simulink library "lib_FDM"  (R2019b)
settings: Solver=VariableStepAuto  StartTime=0.0  StopTime=10.0  RelTol=1e-3
values from neighbouring files (symbols this model uses):
  d = config.d_m    [computeTF.m]
undefined symbols (not defined in the file or in its folder): c_b_WGS, c_flat, c_grav, c_rot, c_rsma, Cd0, Cdcl, Cdcl2, Cl0, Cla, Cld, Cma, Cmd, Cmq, Cnb, Cnd, Cnr, Cra, Crd, Crp, Cy0, Cyb, Cyd, dmdt, Earth, HIL_Data, InitThrust, launchPos, me, mf, mp, Sref, tb, TF, theta0, WGS84
libraries: simulink_extras x14, $bdroot x7, simulink x5, lib_Fin_Deflections x3, aerolibasang x2, sharedtransform x1, aerolibtransform2 x1, aerolibbdyn x1, aerolibatmos2 x1, aerolibutil x1, aerolib6dof2 x1
(part 6 of 8)

== system lib_FDM/FDM/FDM_Sophisticated/environment/atmosphere_static_ISO_2533/tmp_and_pressure_ISO_2533/static_Temperature ==
  Tmp_ref : Inport
  h_geop : Inport  Port=2
  h_geop_ref : Inport  Port=3
  Add : Sum
  Product : Product
  Subtract : Sum  Inputs=+-
  Tmp_gradient_tropo : Constant  Value=HIL_Data.FDM.soph.bus2.c_be
  Tmp : Outport  VectorParamsAs1DForOutWhenUnconnected=off
  wires:
  h_geop_ref/1 -> Subtract/2
  h_geop/1 -> Subtract/1
  Tmp_ref/1 -> Add/1
  Add/1 -> Tmp/1  "Tmp"
  Product/1 -> Add/2
  Tmp_gradient_tropo/1 -> Product/1
  Subtract/1 -> Product/2

== system lib_FDM/FDM/FDM_Sophisticated/environment/atmosphere_static_ISO_2533/tmp_and_pressure_ISO_2533/static_pressure ==
  h_geop_ref : Inport
  h_geop : Inport  Port=2
  Tmp_ref : Inport  Port=3
  pa_ref : Inport  Port=4
  Add : Sum
  Constant1 : Constant
  Divide : Product  Inputs=*/*
  Math Function : Math  Operator=pow  SaturateOnIntegerOverflow=on
  Product : Product
  Subtract : Sum  Inputs=-+
  Tmp_gradient_tropo : Constant  Value=HIL_Data.FDM.soph.bus2.c_be
  pressure_exponent : Constant  Value=HIL_Data.FDM.soph.bus2.c_pe
  pa : Outport  VectorParamsAs1DForOutWhenUnconnected=off
  wires:
  Tmp_gradient_tropo/1 -> Divide/3
  Product/1 -> pa/1  "pa"
  Constant1/1 -> Add/1
  Subtract/1 -> Divide/1
  Math Function/1 -> Product/1
  pa_ref/1 -> Product/2
  Add/1 -> Math Function/1
  Tmp_ref/1 -> Divide/2
  h_geop_ref/1 -> Subtract/1
  Divide/1 -> Add/2
  h_geop/1 -> Subtract/2
  pressure_exponent/1 -> Math Function/2

== system lib_FDM/FDM/FDM_Sophisticated/gravity/launch_rail/initial_altitude/trafo_E_to_geodetic ==
  note: Inputs [size]:
      |
      | position_E [3]
  note: Outputs [size]:
      |
      | geodetic longitude [1]
      | geodetic latitude [1]
      | geodetic altitude [1]
  pBEE : Inport
  Geodetic_altitude : Subsystem
  Geodetic_latitude : Subsystem
  Selector1 : Selector  IndexMode=Zero-based  InputPortWidth=3  IndexOptions=Index vector (dialog)  Indices=1  OutputSizes=1
  Selector2 : Selector  IndexMode=Zero-based  InputPortWidth=3  IndexOptions=Index vector (dialog)  Indices=0  OutputSizes=1
  Trigonometric Function1 : Trigonometry  Operator=atan2
  c_flat : Constant  Value=c_flat
  c_rsma : Constant  Value=c_rsma
  lon : Outport  VectorParamsAs1DForOutWhenUnconnected=off
  lat : Outport  Port=2  VectorParamsAs1DForOutWhenUnconnected=off
  alt : Outport  Port=3  VectorParamsAs1DForOutWhenUnconnected=off
  wires:
  pBEE/1 -> Geodetic_altitude/1(pBEE), Geodetic_latitude/1(pBEE), Selector2/1, Selector1/1  "pBEE"
  Trigonometric Function1/1 -> lon/1  "lon"
  Geodetic_altitude/1(alt) -> alt/1
  Geodetic_latitude/1(lat) -> lat/1, Geodetic_altitude/4(lat)
  Selector2/1 -> Trigonometric Function1/2  "pBEE_x"
  Selector1/1 -> Trigonometric Function1/1  "pBEE_y"
  c_rsma/1 -> Geodetic_altitude/2(c_rsma), Geodetic_latitude/2(c_rsma)  "c_rsma"
  c_flat/1 -> Geodetic_latitude/3(c_flat), Geodetic_altitude/3(c_flat)  "c_flat"

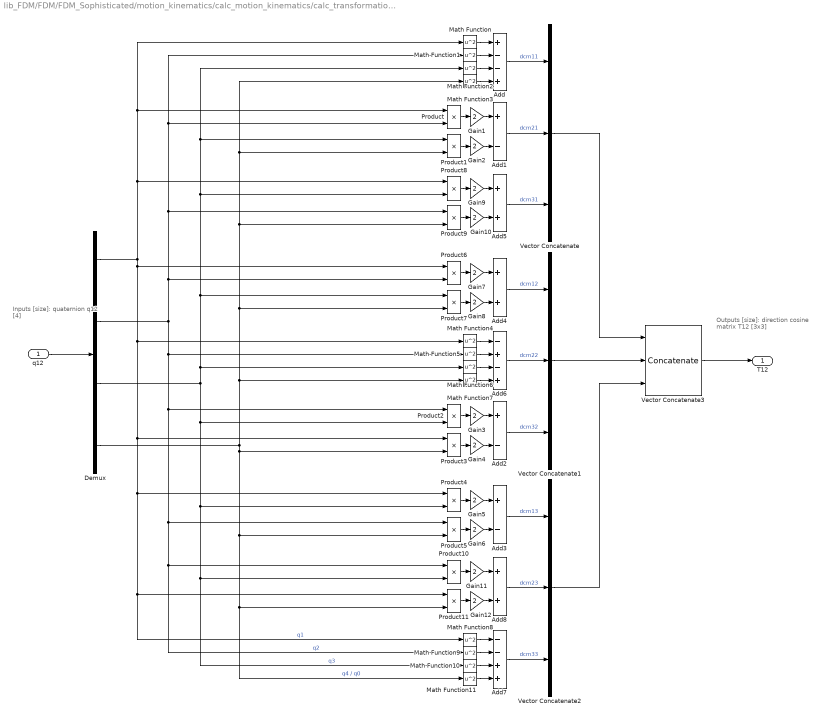
== system lib_FDM/FDM/FDM_Sophisticated/motion_kinematics/calc_motion_kinematics/calc_transformation_matrix/T12_from_q1 ==
  note: Outputs [size]:
      |
      | direction cosine matrix T12 [3x3]
  note: Inputs [size]:
      |
      | quaternion q12 [4]
  q12 : Inport  PortDimensions=4
  Add : Sum  Inputs=+--+
  Add1 : Sum  Inputs=+-
  Add2 : Sum  Inputs=+-
  Add3 : Sum  Inputs=+-
  Add4 : Sum
  Add5 : Sum
  Add6 : Sum  Inputs=-+-+
  Add7 : Sum  Inputs=--++
  Add8 : Sum
  Demux : Demux
  Gain{1..12} (12 alike) : Gain  Gain=2
  Math Function{,1..11} (12 alike) : Math  Operator=square  SaturateOnIntegerOverflow=on
  Product{,1..11} (12 alike) : Product
  Vector Concatenate : Concatenate  NumInputs=3
  Vector Concatenate1 : Concatenate  NumInputs=3
  Vector Concatenate2 : Concatenate  NumInputs=3
  Vector Concatenate3 : Concatenate  NumInputs=3  Mode=Multidimensional array  ConcatenateDimension=2
  T12 : Outport  PortDimensions=[3 3]  VectorParamsAs1DForOutWhenUnconnected=off
  wires:
  q12/1 -> Demux/1
  Demux/1 -> Product8/1, Product/1, Math Function/1, Product3/1, Product4/1, Product11/1, Math Function8/1, Math Function4/1, Product6/1  "q1"
  Demux/2 -> Product2/1, Product5/1, Product10/1, Math Function9/1, Math Function5/1, Product6/2, Product9/1, Product/2, Math Function1/1  "q2"
  Demux/3 -> Product2/2, Product4/2, Math Function10/1, Product10/2, Math Function6/1, Product7/1, Product8/2, Product1/1, Math Function2/1  "q3"
  Demux/4 -> Math Function7/1, Product7/2, Product9/2, Product1/2, Math Function3/1, Product5/2, Math Function11/1, Product11/2, Product3/2  "q4 / q0"
  Vector Concatenate3/1 -> T12/1
  Vector Concatenate/1 -> Vector Concatenate3/1
  Vector Concatenate2/1 -> Vector Concatenate3/3
  Vector Concatenate1/1 -> Vector Concatenate3/2
  Add/1 -> Vector Concatenate/1  "dcm11"
  Add1/1 -> Vector Concatenate/2  "dcm21"
  Add5/1 -> Vector Concatenate/3  "dcm31"
  Add4/1 -> Vector Concatenate1/1  "dcm12"
  Add6/1 -> Vector Concatenate1/2  "dcm22"
  Add2/1 -> Vector Concatenate1/3  "dcm32"
  Add3/1 -> Vector Concatenate2/1  "dcm13"
  Add8/1 -> Vector Concatenate2/2  "dcm23"
  Add7/1 -> Vector Concatenate2/3  "dcm33"
  Math Function/1 -> Add/1
  Math Function1/1 -> Add/2
  Math Function2/1 -> Add/3
  Math Function3/1 -> Add/4
  Product/1 -> Gain1/1
  Product1/1 -> Gain2/1
  Gain1/1 -> Add1/1
  Gain2/1 -> Add1/2
  Gain4/1 -> Add2/2
  Gain3/1 -> Add2/1
  Product3/1 -> Gain4/1
  Product2/1 -> Gain3/1
  Gain6/1 -> Add3/2
  Gain5/1 -> Add3/1
  Product5/1 -> Gain6/1
  Product4/1 -> Gain5/1
  Gain8/1 -> Add4/2
  Gain7/1 -> Add4/1
  Product7/1 -> Gain8/1
  Product6/1 -> Gain7/1
  Gain10/1 -> Add5/2
  Gain9/1 -> Add5/1
  Product9/1 -> Gain10/1
  Product8/1 -> Gain9/1
  Math Function6/1 -> Add6/3
  Math Function7/1 -> Add6/4
  Math Function5/1 -> Add6/2
  Math Function4/1 -> Add6/1
  Math Function10/1 -> Add7/3
  Math Function11/1 -> Add7/4
  Math Function9/1 -> Add7/2
  Math Function8/1 -> Add7/1
  Gain12/1 -> Add8/2
  Gain11/1 -> Add8/1
  Product11/1 -> Gain12/1
  Product10/1 -> Gain11/1

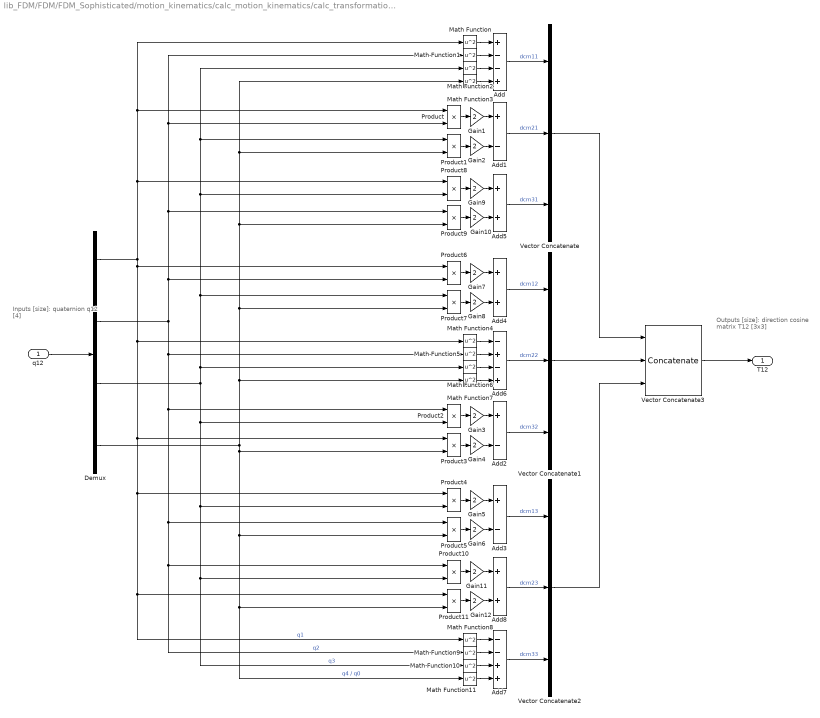
== system lib_FDM/FDM/FDM_Sophisticated/motion_kinematics/calc_motion_kinematics/calc_transformation_matrix/T12_from_q12 ==
  note: Outputs [size]:
      |
      | direction cosine matrix T12 [3x3]
  note: Inputs [size]:
      |
      | quaternion q12 [4]
  q12 : Inport  PortDimensions=4
  Add : Sum  Inputs=+--+
  Add1 : Sum  Inputs=+-
  Add2 : Sum  Inputs=+-
  Add3 : Sum  Inputs=+-
  Add4 : Sum
  Add5 : Sum
  Add6 : Sum  Inputs=-+-+
  Add7 : Sum  Inputs=--++
  Add8 : Sum
  Demux : Demux
  Gain{1..12} (12 alike) : Gain  Gain=2
  Math Function{,1..11} (12 alike) : Math  Operator=square  SaturateOnIntegerOverflow=on
  Product{,1..11} (12 alike) : Product
  Vector Concatenate : Concatenate  NumInputs=3
  Vector Concatenate1 : Concatenate  NumInputs=3
  Vector Concatenate2 : Concatenate  NumInputs=3
  Vector Concatenate3 : Concatenate  NumInputs=3  Mode=Multidimensional array  ConcatenateDimension=2
  T12 : Outport  PortDimensions=[3 3]  VectorParamsAs1DForOutWhenUnconnected=off
  wires:
  q12/1 -> Demux/1
  Demux/1 -> Product8/1, Product/1, Math Function/1, Product3/1, Product4/1, Product11/1, Math Function8/1, Math Function4/1, Product6/1  "q1"
  Demux/2 -> Product2/1, Product5/1, Product10/1, Math Function9/1, Math Function5/1, Product6/2, Product9/1, Product/2, Math Function1/1  "q2"
  Demux/3 -> Product2/2, Product4/2, Math Function10/1, Product10/2, Math Function6/1, Product7/1, Product8/2, Product1/1, Math Function2/1  "q3"
  Demux/4 -> Math Function7/1, Product7/2, Product9/2, Product1/2, Math Function3/1, Product5/2, Math Function11/1, Product11/2, Product3/2  "q4 / q0"
  Vector Concatenate3/1 -> T12/1
  Vector Concatenate/1 -> Vector Concatenate3/1
  Vector Concatenate2/1 -> Vector Concatenate3/3
  Vector Concatenate1/1 -> Vector Concatenate3/2
  Add/1 -> Vector Concatenate/1  "dcm11"
  Add1/1 -> Vector Concatenate/2  "dcm21"
  Add5/1 -> Vector Concatenate/3  "dcm31"
  Add4/1 -> Vector Concatenate1/1  "dcm12"
  Add6/1 -> Vector Concatenate1/2  "dcm22"
  Add2/1 -> Vector Concatenate1/3  "dcm32"
  Add3/1 -> Vector Concatenate2/1  "dcm13"
  Add8/1 -> Vector Concatenate2/2  "dcm23"
  Add7/1 -> Vector Concatenate2/3  "dcm33"
  Math Function/1 -> Add/1
  Math Function1/1 -> Add/2
  Math Function2/1 -> Add/3
  Math Function3/1 -> Add/4
  Product/1 -> Gain1/1
  Product1/1 -> Gain2/1
  Gain1/1 -> Add1/1
  Gain2/1 -> Add1/2
  Gain4/1 -> Add2/2
  Gain3/1 -> Add2/1
  Product3/1 -> Gain4/1
  Product2/1 -> Gain3/1
  Gain6/1 -> Add3/2
  Gain5/1 -> Add3/1
  Product5/1 -> Gain6/1
  Product4/1 -> Gain5/1
  Gain8/1 -> Add4/2
  Gain7/1 -> Add4/1
  Product7/1 -> Gain8/1
  Product6/1 -> Gain7/1
  Gain10/1 -> Add5/2
  Gain9/1 -> Add5/1
  Product9/1 -> Gain10/1
  Product8/1 -> Gain9/1
  Math Function6/1 -> Add6/3
  Math Function7/1 -> Add6/4
  Math Function5/1 -> Add6/2
  Math Function4/1 -> Add6/1
  Math Function10/1 -> Add7/3
  Math Function11/1 -> Add7/4
  Math Function9/1 -> Add7/2
  Math Function8/1 -> Add7/1
  Gain12/1 -> Add8/2
  Gain11/1 -> Add8/1
  Product11/1 -> Gain12/1
  Product10/1 -> Gain11/1

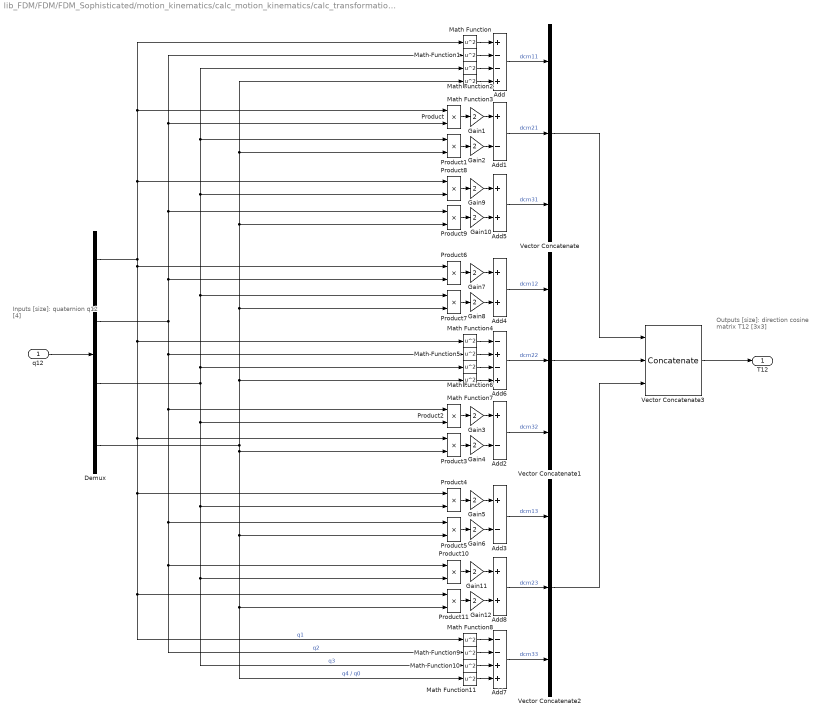
== system lib_FDM/FDM/FDM_Sophisticated/motion_kinematics/calc_motion_kinematics/calc_transformation_matrix/T12_from_q2 ==
  note: Outputs [size]:
      |
      | direction cosine matrix T12 [3x3]
  note: Inputs [size]:
      |
      | quaternion q12 [4]
  q12 : Inport  PortDimensions=4
  Add : Sum  Inputs=+--+
  Add1 : Sum  Inputs=+-
  Add2 : Sum  Inputs=+-
  Add3 : Sum  Inputs=+-
  Add4 : Sum
  Add5 : Sum
  Add6 : Sum  Inputs=-+-+
  Add7 : Sum  Inputs=--++
  Add8 : Sum
  Demux : Demux
  Gain{1..12} (12 alike) : Gain  Gain=2
  Math Function{,1..11} (12 alike) : Math  Operator=square  SaturateOnIntegerOverflow=on
  Product{,1..11} (12 alike) : Product
  Vector Concatenate : Concatenate  NumInputs=3
  Vector Concatenate1 : Concatenate  NumInputs=3
  Vector Concatenate2 : Concatenate  NumInputs=3
  Vector Concatenate3 : Concatenate  NumInputs=3  Mode=Multidimensional array  ConcatenateDimension=2
  T12 : Outport  PortDimensions=[3 3]  VectorParamsAs1DForOutWhenUnconnected=off
  wires:
  q12/1 -> Demux/1
  Demux/1 -> Product8/1, Product/1, Math Function/1, Product3/1, Product4/1, Product11/1, Math Function8/1, Math Function4/1, Product6/1  "q1"
  Demux/2 -> Product2/1, Product5/1, Product10/1, Math Function9/1, Math Function5/1, Product6/2, Product9/1, Product/2, Math Function1/1  "q2"
  Demux/3 -> Product2/2, Product4/2, Math Function10/1, Product10/2, Math Function6/1, Product7/1, Product8/2, Product1/1, Math Function2/1  "q3"
  Demux/4 -> Math Function7/1, Product7/2, Product9/2, Product1/2, Math Function3/1, Product5/2, Math Function11/1, Product11/2, Product3/2  "q4 / q0"
  Vector Concatenate3/1 -> T12/1
  Vector Concatenate/1 -> Vector Concatenate3/1
  Vector Concatenate2/1 -> Vector Concatenate3/3
  Vector Concatenate1/1 -> Vector Concatenate3/2
  Add/1 -> Vector Concatenate/1  "dcm11"
  Add1/1 -> Vector Concatenate/2  "dcm21"
  Add5/1 -> Vector Concatenate/3  "dcm31"
  Add4/1 -> Vector Concatenate1/1  "dcm12"
  Add6/1 -> Vector Concatenate1/2  "dcm22"
  Add2/1 -> Vector Concatenate1/3  "dcm32"
  Add3/1 -> Vector Concatenate2/1  "dcm13"
  Add8/1 -> Vector Concatenate2/2  "dcm23"
  Add7/1 -> Vector Concatenate2/3  "dcm33"
  Math Function/1 -> Add/1
  Math Function1/1 -> Add/2
  Math Function2/1 -> Add/3
  Math Function3/1 -> Add/4
  Product/1 -> Gain1/1
  Product1/1 -> Gain2/1
  Gain1/1 -> Add1/1
  Gain2/1 -> Add1/2
  Gain4/1 -> Add2/2
  Gain3/1 -> Add2/1
  Product3/1 -> Gain4/1
  Product2/1 -> Gain3/1
  Gain6/1 -> Add3/2
  Gain5/1 -> Add3/1
  Product5/1 -> Gain6/1
  Product4/1 -> Gain5/1
  Gain8/1 -> Add4/2
  Gain7/1 -> Add4/1
  Product7/1 -> Gain8/1
  Product6/1 -> Gain7/1
  Gain10/1 -> Add5/2
  Gain9/1 -> Add5/1
  Product9/1 -> Gain10/1
  Product8/1 -> Gain9/1
  Math Function6/1 -> Add6/3
  Math Function7/1 -> Add6/4
  Math Function5/1 -> Add6/2
  Math Function4/1 -> Add6/1
  Math Function10/1 -> Add7/3
  Math Function11/1 -> Add7/4
  Math Function9/1 -> Add7/2
  Math Function8/1 -> Add7/1
  Gain12/1 -> Add8/2
  Gain11/1 -> Add8/1
  Product11/1 -> Gain12/1
  Product10/1 -> Gain11/1

== system lib_FDM/FDM/FDM_Sophisticated/motion_kinematics/calc_motion_kinematics/calc_transformation_matrix/conjugate_quaternion ==
  note: Inputs [size]:
      |
      | q [4]
  note: Outputs [size]:
      |
      | q_conj [4]
  q : Inport
  Demux : Demux  Outputs=[3;1]
  Gain1 : Gain  Gain=-1
  Vector Concatenate : Concatenate
  q_conj : Outport  VectorParamsAs1DForOutWhenUnconnected=off
  wires:
  q/1 -> Demux/1
  Vector Concatenate/1 -> q_conj/1
  Demux/1 -> Gain1/1
  Gain1/1 -> Vector Concatenate/1
  Demux/2 -> Vector Concatenate/2

== system lib_FDM/FDM/FDM_Sophisticated/motion_kinematics/calc_motion_kinematics/calc_transformation_matrix/q31_from_q32_mul_q1 ==
  note: Inputs [size]:
      |
      | quaternion q32 [4]
      | quaternion q21 [4]
  note: Outputs [size]:
      |
      | quaternion q31 [4]
  q32 : Inport
  q21 : Inport  Port=2
  Add : Sum  Inputs=++++
  Constant : Constant
  Constant1 : Constant  Value=-1
  Demux1 : Demux
  Product{,1..4} (5 alike) : Product
  Product8 : Product  Multiplication=Matrix(*)
  Q_1 : Constant  Value=[0 0 0 1; 0 0 1 0; 0 -1 0 0; -1 0 0 0]
  Q_2 : Constant  Value=[0 0 -1 0; 0 0 0 1; 1 0 0 0; 0 -1 0 0]
  Q_3 : Constant  Value=[0 1 0 0; -1 0 0 0; 0 0 0 1; 0 0 -1 0]
  Q_4 : Constant  Value=[1 0 0 0; 0 1 0 0; 0 0 1 0; 0 0 0 1]
  Selector : Selector  IndexMode=Zero-based  InputPortWidth=4  IndexOptions=Index vector (dialog)  Indices=3  OutputSizes=1
  Switch : Switch
  normalize_quaternion : Subsystem
      mask help: normalize a quaternion
      mask Help:
      | Name:
      | 
      |     normalize_quaternion
      | 
      | Description:
      | 
      |     This block normalizes the quaternion q21. It should be used as a
      |     safety measure when computing quaternions.
      | 
      | Inputs  [size] [data type] [unit]:
      | 
      |     attitude quaternion q21  [4] [double] [-]
      | 
      | Outputs  [size] [data type] [unit]:
      | 
      |     normalized attitude quaternion q21  [4] [double] [-]
      mask Display: disp (' norm(q)')
  q31 : Outport  VectorParamsAs1DForOutWhenUnconnected=off
  wires:
  q21/1 -> Product8/2
  Demux1/1 -> Product/2  "q1"
  Demux1/2 -> Product1/2  "q2"
  Demux1/3 -> Product2/2  "q3"
  Demux1/4 -> Product3/2  "q4"
  Q_1/1 -> Product/1
  Q_2/1 -> Product1/1
  Q_3/1 -> Product2/1
  Q_4/1 -> Product3/1
  Product/1 -> Add/1
  Product1/1 -> Add/2
  Product2/1 -> Add/3
  Product3/1 -> Add/4
  Add/1 -> Product8/1  "Q(q32)"
  q32/1 -> Demux1/1
  Product8/1 -> normalize_quaternion/1(q)
  normalize_quaternion/1(q_normalized) -> Product4/1, Selector/1
  Selector/1 -> Switch/2
  Product4/1 -> q31/1
  Constant1/1 -> Switch/3
  Constant/1 -> Switch/1
  Switch/1 -> Product4/2

== system lib_FDM/FDM/FDM_Sophisticated/motion_kinematics/calc_motion_kinematics/calc_transformation_matrix/q31_from_q32_mul_q2 ==
  note: Inputs [size]:
      |
      | quaternion q32 [4]
      | quaternion q21 [4]
  note: Outputs [size]:
      |
      | quaternion q31 [4]
  q32 : Inport
  q21 : Inport  Port=2
  Add : Sum  Inputs=++++
  Constant : Constant
  Constant1 : Constant  Value=-1
  Demux1 : Demux
  Product{,1..4} (5 alike) : Product
  Product8 : Product  Multiplication=Matrix(*)
  Q_1 : Constant  Value=[0 0 0 1; 0 0 1 0; 0 -1 0 0; -1 0 0 0]
  Q_2 : Constant  Value=[0 0 -1 0; 0 0 0 1; 1 0 0 0; 0 -1 0 0]
  Q_3 : Constant  Value=[0 1 0 0; -1 0 0 0; 0 0 0 1; 0 0 -1 0]
  Q_4 : Constant  Value=[1 0 0 0; 0 1 0 0; 0 0 1 0; 0 0 0 1]
  Selector : Selector  IndexMode=Zero-based  InputPortWidth=4  IndexOptions=Index vector (dialog)  Indices=3  OutputSizes=1
  Switch : Switch
  normalize_quaternion : Subsystem
      mask help: normalize a quaternion
      mask Help:
      | Name:
      | 
      |     normalize_quaternion
      | 
      | Description:
      | 
      |     This block normalizes the quaternion q21. It should be used as a
      |     safety measure when computing quaternions.
      | 
      | Inputs  [size] [data type] [unit]:
      | 
      |     attitude quaternion q21  [4] [double] [-]
      | 
      | Outputs  [size] [data type] [unit]:
      | 
      |     normalized attitude quaternion q21  [4] [double] [-]
      mask Display: disp (' norm(q)')
  q31 : Outport  VectorParamsAs1DForOutWhenUnconnected=off
  wires:
  q21/1 -> Product8/2
  Demux1/1 -> Product/2  "q1"
  Demux1/2 -> Product1/2  "q2"
  Demux1/3 -> Product2/2  "q3"
  Demux1/4 -> Product3/2  "q4"
  Q_1/1 -> Product/1
  Q_2/1 -> Product1/1
  Q_3/1 -> Product2/1
  Q_4/1 -> Product3/1
  Product/1 -> Add/1
  Product1/1 -> Add/2
  Product2/1 -> Add/3
  Product3/1 -> Add/4
  Add/1 -> Product8/1  "Q(q32)"
  q32/1 -> Demux1/1
  Product8/1 -> normalize_quaternion/1(q)
  normalize_quaternion/1(q_normalized) -> Product4/1, Selector/1
  Selector/1 -> Switch/2
  Product4/1 -> q31/1
  Constant1/1 -> Switch/3
  Constant/1 -> Switch/1
  Switch/1 -> Product4/2

== system lib_FDM/FDM/FDM_Sophisticated/motion_kinematics/calc_motion_kinematics/calc_transformation_matrix/q31_from_q32_mul_q21 ==
  note: Inputs [size]:
      |
      | quaternion q32 [4]
      | quaternion q21 [4]
  note: Outputs [size]:
      |
      | quaternion q31 [4]
  q32 : Inport
  q21 : Inport  Port=2
  Add : Sum  Inputs=++++
  Constant : Constant
  Constant1 : Constant  Value=-1
  Demux1 : Demux
  Product{,1..4} (5 alike) : Product
  Product8 : Product  Multiplication=Matrix(*)
  Q_1 : Constant  Value=[0 0 0 1; 0 0 1 0; 0 -1 0 0; -1 0 0 0]
  Q_2 : Constant  Value=[0 0 -1 0; 0 0 0 1; 1 0 0 0; 0 -1 0 0]
  Q_3 : Constant  Value=[0 1 0 0; -1 0 0 0; 0 0 0 1; 0 0 -1 0]
  Q_4 : Constant  Value=[1 0 0 0; 0 1 0 0; 0 0 1 0; 0 0 0 1]
  Selector : Selector  IndexMode=Zero-based  InputPortWidth=4  IndexOptions=Index vector (dialog)  Indices=3  OutputSizes=1
  Switch : Switch
  normalize_quaternion : Subsystem
      mask help: normalize a quaternion
      mask Help:
      | Name:
      | 
      |     normalize_quaternion
      | 
      | Description:
      | 
      |     This block normalizes the quaternion q21. It should be used as a
      |     safety measure when computing quaternions.
      | 
      | Inputs  [size] [data type] [unit]:
      | 
      |     attitude quaternion q21  [4] [double] [-]
      | 
      | Outputs  [size] [data type] [unit]:
      | 
      |     normalized attitude quaternion q21  [4] [double] [-]
      mask Display: disp (' norm(q)')
  q31 : Outport  VectorParamsAs1DForOutWhenUnconnected=off
  wires:
  q21/1 -> Product8/2
  Demux1/1 -> Product/2  "q1"
  Demux1/2 -> Product1/2  "q2"
  Demux1/3 -> Product2/2  "q3"
  Demux1/4 -> Product3/2  "q4"
  Q_1/1 -> Product/1
  Q_2/1 -> Product1/1
  Q_3/1 -> Product2/1
  Q_4/1 -> Product3/1
  Product/1 -> Add/1
  Product1/1 -> Add/2
  Product2/1 -> Add/3
  Product3/1 -> Add/4
  Add/1 -> Product8/1  "Q(q32)"
  q32/1 -> Demux1/1
  Product8/1 -> normalize_quaternion/1(q)
  normalize_quaternion/1(q_normalized) -> Product4/1, Selector/1
  Selector/1 -> Switch/2
  Product4/1 -> q31/1
  Constant1/1 -> Switch/3
  Constant/1 -> Switch/1
  Switch/1 -> Product4/2

== system lib_FDM/FDM/FDM_Sophisticated/motion_kinematics/calc_motion_kinematics/earth_rotation/earth_rotation_rate ==
  Constant6 : Constant  Value=0
  Constant7 : Constant  Value=HIL_Data.FDM.soph.bus2.c_rot
  Constant8 : Constant  Value=0
  Constant9 : Constant  Value=HIL_Data.FDM.soph.bus2.flag_I_rot
  Switch : Switch  Criteria=u2 > Threshold
  Vector Concatenate : Concatenate  NumInputs=3
  Vector Concatenate1 : Concatenate  NumInputs=3
  wIEE : Outport  VectorParamsAs1DForOutWhenUnconnected=off
  wires:
  Constant8/1 -> Vector Concatenate1/2, Vector Concatenate1/3, Vector Concatenate1/1
  Vector Concatenate1/1 -> Switch/3  "wIEE"
  Constant7/1 -> Vector Concatenate/3
  Vector Concatenate/1 -> Switch/1  "wIEE"
  Constant9/1 -> Switch/2
  Constant6/1 -> Vector Concatenate/1, Vector Concatenate/2
  Switch/1 -> wIEE/1  "wIEE"

== system lib_FDM/FDM/FDM_Sophisticated/motion_kinematics/calc_motion_kinematics/earth_rotation/quaternion_integration ==
  wEIE : Inport
  Constant8 : Constant  Value=HIL_Data.FDM.soph.bus2.qIE_0
  Subsystem1 : Subsystem
  T12_from_q12 : Subsystem
      mask help: Transforms a quaternion into a Direction Cosine Matrix
      mask Help:
      | Name:
      | 
      |     T12_from_q12
      | 
      | Description:
      | 
      |     This block implements the transformation of a quaternion into the
      |     corresponding direction cosine matrix DCM.
      | 
      | Inputs  [size] [data type] [unit]:
      | 
      |     quaternion q12 [4] [double] [-]
      | 
      | Outputs  [size] [data type] [unit]:
      | 
      |     direction cosine matrix T12  [3x3] [double] [-]
      mask Display:
      | %port_label('input', 1, 'q12')
      | %port_label('output', 1, 'T12')
      | disp('q \rightarrow DCM','texmode','on')
  integration_eom : Integrator  InitialConditionSource=external
  qIE : Outport  VectorParamsAs1DForOutWhenUnconnected=off
  TIE : Outport  Port=2  VectorParamsAs1DForOutWhenUnconnected=off
  wires:
  Constant8/1 -> integration_eom/2
  T12_from_q12/1(T12) -> TIE/1  "TIE"
  wEIE/1 -> Subsystem1/1(wEIE)
  integration_eom/1 -> T12_from_q12/1(q12), Subsystem1/2(qIE), qIE/1  "qIE"
  Subsystem1/1(d_qIE) -> integration_eom/1

== system lib_FDM/FDM/FDM_Sophisticated/motion_kinematics/calc_motion_kinematics/earth_rotation/quaternion_integration1 ==
  wGEG : Inport
  Constant8 : Constant  Value=HIL_Data.FDM.soph.bus2.qEG_0
  Subsystem1 : Subsystem
  T12_from_q12 : Subsystem
      mask help: Transforms a quaternion into a Direction Cosine Matrix
      mask Help:
      | Name:
      | 
      |     T12_from_q12
      | 
      | Description:
      | 
      |     This block implements the transformation of a quaternion into the
      |     corresponding direction cosine matrix DCM.
      | 
      | Inputs  [size] [data type] [unit]:
      | 
      |     quaternion q12 [4] [double] [-]
      | 
      | Outputs  [size] [data type] [unit]:
      | 
      |     direction cosine matrix T12  [3x3] [double] [-]
      mask Display:
      | %port_label('input', 1, 'q12')
      | %port_label('output', 1, 'T12')
      | disp('q \rightarrow DCM','texmode','on')
  integration_eom : Integrator  InitialConditionSource=external
  qEG : Outport  VectorParamsAs1DForOutWhenUnconnected=off
  TEG : Outport  Port=2  VectorParamsAs1DForOutWhenUnconnected=off
  wires:
  Subsystem1/1(d_qEG) -> integration_eom/1
  integration_eom/1 -> qEG/1, Subsystem1/2(qEG), T12_from_q12/1(q12)  "qEG"
  wGEG/1 -> Subsystem1/1(wGEG)
  T12_from_q12/1(T12) -> TEG/1  "TEG"
  Constant8/1 -> integration_eom/2

== system lib_FDM/FDM/FDM_Sophisticated/motion_kinematics/calc_motion_kinematics/earth_rotation/transport_rate ==
  lat : Inport
  lon : Inport  Port=2
  Constant8 : Constant  Value=0
  Constant9 : Constant  Value=HIL_Data.FDM.soph.bus2.flag_I_flat
  Derivative : Derivative  CoefficientInTFapproximation=1
  Derivative1 : Derivative  CoefficientInTFapproximation=1
  Gain1 : Gain  Gain=-1
  Gain2 : Gain  Gain=-1
  Product : Product
  Product1 : Product
  Switch : Switch  Criteria=u2 > Threshold
  Trigonometric Function : Trigonometry
  Trigonometric Function1 : Trigonometry  Operator=cos
  Vector Concatenate : Concatenate  NumInputs=3
  Vector Concatenate1 : Concatenate  NumInputs=3
  wEGG : Outport  VectorParamsAs1DForOutWhenUnconnected=off
  wires:
  Switch/1 -> wEGG/1  "wEGG"
  Constant8/1 -> Vector Concatenate1/2, Vector Concatenate1/3, Vector Concatenate1/1
  Vector Concatenate1/1 -> Switch/1  "wEGG"
  Constant9/1 -> Switch/2
  Vector Concatenate/1 -> Switch/3  "wEGG"
  lon/1 -> Derivative1/1
  Trigonometric Function1/1 -> Product1/2
  Product1/1 -> Vector Concatenate/1
  Gain1/1 -> Vector Concatenate/2
  Gain2/1 -> Vector Concatenate/3
  Product/1 -> Gain2/1
  Derivative1/1 -> Product/2, Product1/1
  lat/1 -> Trigonometric Function/1, Derivative/1, Trigonometric Function1/1
  Trigonometric Function/1 -> Product/1
  Derivative/1 -> Gain1/1

== system lib_FDM/FDM/FDM_Sophisticated/propulsion/prp_uncertainty/3_rot_mat/1. Rotation x-Achse ==
  alpha1 : Inport
  Constant : Constant
  Constant{1..2,7..8} (4 alike) : Constant  Value=0
  Gain : Gain  Gain=-1
  Matrix Concatenate : Concatenate  NumInputs=3  Mode=Multidimensional array  ConcatenateDimension=2
  Mux : Mux  Inputs=3
  Mux1 : Mux  Inputs=3
  Mux2 : Mux  Inputs=3
  Trigonometric Function : Trigonometry  Operator=cos
  Trigonometric Function1 : Trigonometry
  Trigonometric Function2 : Trigonometry
  Trigonometric Function3 : Trigonometry  Operator=cos
  1Rot_Matrix_x : Outport  VectorParamsAs1DForOutWhenUnconnected=off
  wires:
  Matrix Concatenate/1 -> 1Rot_Matrix_x/1
  Mux2/1 -> Matrix Concatenate/3
  Mux1/1 -> Matrix Concatenate/2
  Mux/1 -> Matrix Concatenate/1
  Trigonometric Function3/1 -> Mux2/3
  Trigonometric Function1/1 -> Mux2/2
  Constant7/1 -> Mux2/1
  Trigonometric Function2/1 -> Gain/1
  Trigonometric Function/1 -> Mux1/2
  Constant8/1 -> Mux1/1
  Constant2/1 -> Mux/3
  Constant1/1 -> Mux/2
  Constant/1 -> Mux/1
  alpha1/1 -> Trigonometric Function3/1, Trigonometric Function1/1, Trigonometric Function/1, Trigonometric Function2/1
  Gain/1 -> Mux1/3

== system lib_FDM/FDM/FDM_Sophisticated/propulsion/prp_uncertainty/3_rot_mat/1. Rotation y-Achse ==
  alpha1 : Inport
  Constant{,2,7..8} (4 alike) : Constant  Value=0
  Constant1 : Constant
  Gain1 : Gain  Gain=-1
  Matrix Concatenate : Concatenate  NumInputs=3  Mode=Multidimensional array  ConcatenateDimension=2
  Mux : Mux  Inputs=3
  Mux1 : Mux  Inputs=3
  Mux2 : Mux  Inputs=3
  Trigonometric Function : Trigonometry  Operator=cos
  Trigonometric Function1 : Trigonometry
  Trigonometric Function2 : Trigonometry
  Trigonometric Function3 : Trigonometry  Operator=cos
  1Rot_Matrix_y : Outport  VectorParamsAs1DForOutWhenUnconnected=off
  wires:
  Matrix Concatenate/1 -> 1Rot_Matrix_y/1
  Constant7/1 -> Mux2/2
  Trigonometric Function2/1 -> Mux/3
  Trigonometric Function/1 -> Mux/1
  Constant8/1 -> Mux/2
  alpha1/1 -> Trigonometric Function/1, Trigonometric Function2/1, Trigonometric Function3/1, Trigonometric Function1/1
  Constant/1 -> Mux1/1
  Constant1/1 -> Mux1/2
  Constant2/1 -> Mux1/3
  Trigonometric Function1/1 -> Gain1/1
  Trigonometric Function3/1 -> Mux2/3
  Mux/1 -> Matrix Concatenate/1
  Mux1/1 -> Matrix Concatenate/2
  Mux2/1 -> Matrix Concatenate/3
  Gain1/1 -> Mux2/1

== system lib_FDM/FDM/FDM_Sophisticated/propulsion/prp_uncertainty/3_rot_mat/1. Rotation z-Achse ==
  alpha1 : Inport
  Constant{4,7..8,10} (4 alike) : Constant  Value=0
  Constant11 : Constant
  Gain : Gain  Gain=-1
  Matrix Concatenate : Concatenate  NumInputs=3  Mode=Multidimensional array  ConcatenateDimension=2
  Mux : Mux  Inputs=3
  Mux1 : Mux  Inputs=3
  Mux2 : Mux  Inputs=3
  Trigonometric Function : Trigonometry  Operator=cos
  Trigonometric Function1 : Trigonometry
  Trigonometric Function3 : Trigonometry  Operator=cos
  Trigonometric Function4 : Trigonometry
  1Rot_Matrix_z : Outport  VectorParamsAs1DForOutWhenUnconnected=off
  wires:
  alpha1/1 -> Trigonometric Function1/1, Trigonometric Function/1, Trigonometric Function4/1, Trigonometric Function3/1
  Matrix Concatenate/1 -> 1Rot_Matrix_z/1
  Constant8/1 -> Mux/3
  Trigonometric Function4/1 -> Gain/1
  Trigonometric Function3/1 -> Mux/1
  Constant11/1 -> Mux2/3
  Constant10/1 -> Mux2/2
  Constant4/1 -> Mux2/1
  Constant7/1 -> Mux1/3
  Trigonometric Function1/1 -> Mux1/1
  Mux2/1 -> Matrix Concatenate/3
  Mux1/1 -> Matrix Concatenate/2
  Mux/1 -> Matrix Concatenate/1
  Trigonometric Function/1 -> Mux1/2
  Gain/1 -> Mux/2

== system lib_FDM/FDM/FDM_Sophisticated/propulsion/prp_uncertainty/3_rot_mat/2. Rotation x-Achse ==
  alpha2 : Inport
  Constant : Constant
  Constant{1..2,7..8} (4 alike) : Constant  Value=0
  Gain : Gain  Gain=-1
  Matrix Concatenate : Concatenate  NumInputs=3  Mode=Multidimensional array  ConcatenateDimension=2
  Mux : Mux  Inputs=3
  Mux1 : Mux  Inputs=3
  Mux2 : Mux  Inputs=3
  Trigonometric Function : Trigonometry  Operator=cos
  Trigonometric Function1 : Trigonometry
  Trigonometric Function2 : Trigonometry
  Trigonometric Function3 : Trigonometry  Operator=cos
  2Rot_Matrix_x : Outport  VectorParamsAs1DForOutWhenUnconnected=off
  wires:
  Matrix Concatenate/1 -> 2Rot_Matrix_x/1
  Mux2/1 -> Matrix Concatenate/3
  Mux1/1 -> Matrix Concatenate/2
  Mux/1 -> Matrix Concatenate/1
  Trigonometric Function3/1 -> Mux2/3
  Trigonometric Function1/1 -> Mux2/2
  Constant7/1 -> Mux2/1
  Trigonometric Function2/1 -> Gain/1
  Trigonometric Function/1 -> Mux1/2
  Constant8/1 -> Mux1/1
  Constant2/1 -> Mux/3
  Constant1/1 -> Mux/2
  Constant/1 -> Mux/1
  alpha2/1 -> Trigonometric Function3/1, Trigonometric Function1/1, Trigonometric Function/1, Trigonometric Function2/1
  Gain/1 -> Mux1/3

== system lib_FDM/FDM/FDM_Sophisticated/propulsion/prp_uncertainty/3_rot_mat/2. Rotation y-Achse ==
  alpha2 : Inport
  Constant{,2,7..8} (4 alike) : Constant  Value=0
  Constant1 : Constant
  Gain1 : Gain  Gain=-1
  Matrix Concatenate : Concatenate  NumInputs=3  Mode=Multidimensional array  ConcatenateDimension=2
  Mux : Mux  Inputs=3
  Mux1 : Mux  Inputs=3
  Mux2 : Mux  Inputs=3
  Trigonometric Function : Trigonometry  Operator=cos
  Trigonometric Function1 : Trigonometry
  Trigonometric Function2 : Trigonometry
  Trigonometric Function3 : Trigonometry  Operator=cos
  2Rot_Matrix_y : Outport  VectorParamsAs1DForOutWhenUnconnected=off
  wires:
  Matrix Concatenate/1 -> 2Rot_Matrix_y/1
  Constant7/1 -> Mux2/2
  Trigonometric Function2/1 -> Mux/3
  Trigonometric Function/1 -> Mux/1
  Constant8/1 -> Mux/2
  alpha2/1 -> Trigonometric Function/1, Trigonometric Function2/1, Trigonometric Function3/1, Trigonometric Function1/1
  Constant/1 -> Mux1/1
  Constant1/1 -> Mux1/2
  Constant2/1 -> Mux1/3
  Trigonometric Function1/1 -> Gain1/1
  Trigonometric Function3/1 -> Mux2/3
  Mux/1 -> Matrix Concatenate/1
  Mux1/1 -> Matrix Concatenate/2
  Mux2/1 -> Matrix Concatenate/3
  Gain1/1 -> Mux2/1

== system lib_FDM/FDM/FDM_Sophisticated/propulsion/prp_uncertainty/3_rot_mat/2. Rotation z-Achse ==
  alpha2 : Inport
  Constant{4,7..8,10} (4 alike) : Constant  Value=0
  Constant11 : Constant
  Gain : Gain  Gain=-1
  Matrix Concatenate : Concatenate  NumInputs=3  Mode=Multidimensional array  ConcatenateDimension=2
  Mux : Mux  Inputs=3
  Mux1 : Mux  Inputs=3
  Mux2 : Mux  Inputs=3
  Trigonometric Function : Trigonometry  Operator=cos
  Trigonometric Function1 : Trigonometry
  Trigonometric Function3 : Trigonometry  Operator=cos
  Trigonometric Function4 : Trigonometry
  2Rot_Matrix_z : Outport  VectorParamsAs1DForOutWhenUnconnected=off
  wires:
  alpha2/1 -> Trigonometric Function1/1, Trigonometric Function/1, Trigonometric Function4/1, Trigonometric Function3/1
  Matrix Concatenate/1 -> 2Rot_Matrix_z/1
  Constant8/1 -> Mux/3
  Trigonometric Function4/1 -> Gain/1
  Trigonometric Function3/1 -> Mux/1
  Constant11/1 -> Mux2/3
  Constant10/1 -> Mux2/2
  Constant4/1 -> Mux2/1
  Constant7/1 -> Mux1/3
  Trigonometric Function1/1 -> Mux1/1
  Mux2/1 -> Matrix Concatenate/3
  Mux1/1 -> Matrix Concatenate/2
  Mux/1 -> Matrix Concatenate/1
  Trigonometric Function/1 -> Mux1/2
  Gain/1 -> Mux/2

== system lib_FDM/FDM/FDM_Sophisticated/propulsion/prp_uncertainty/3_rot_mat/3. Rotation x-Achse ==
  alpha3 : Inport
  Constant : Constant
  Constant{1..2,7..8} (4 alike) : Constant  Value=0
  Gain : Gain  Gain=-1
  Matrix Concatenate : Concatenate  NumInputs=3  Mode=Multidimensional array  ConcatenateDimension=2
  Mux : Mux  Inputs=3
  Mux1 : Mux  Inputs=3
  Mux2 : Mux  Inputs=3
  Trigonometric Function : Trigonometry  Operator=cos
  Trigonometric Function1 : Trigonometry
  Trigonometric Function2 : Trigonometry
  Trigonometric Function3 : Trigonometry  Operator=cos
  3Rot_Matrix_x : Outport  VectorParamsAs1DForOutWhenUnconnected=off
  wires:
  Matrix Concatenate/1 -> 3Rot_Matrix_x/1
  Mux2/1 -> Matrix Concatenate/3
  Mux1/1 -> Matrix Concatenate/2
  Mux/1 -> Matrix Concatenate/1
  Trigonometric Function3/1 -> Mux2/3
  Trigonometric Function1/1 -> Mux2/2
  Constant7/1 -> Mux2/1
  Trigonometric Function2/1 -> Gain/1
  Trigonometric Function/1 -> Mux1/2
  Constant8/1 -> Mux1/1
  Constant2/1 -> Mux/3
  Constant1/1 -> Mux/2
  Constant/1 -> Mux/1
  alpha3/1 -> Trigonometric Function3/1, Trigonometric Function1/1, Trigonometric Function/1, Trigonometric Function2/1
  Gain/1 -> Mux1/3

== system lib_FDM/FDM/FDM_Sophisticated/propulsion/prp_uncertainty/3_rot_mat/3. Rotation y-Achse ==
  alpha3 : Inport
  Constant{,2,7..8} (4 alike) : Constant  Value=0
  Constant1 : Constant
  Gain1 : Gain  Gain=-1
  Matrix Concatenate : Concatenate  NumInputs=3  Mode=Multidimensional array  ConcatenateDimension=2
  Mux : Mux  Inputs=3
  Mux1 : Mux  Inputs=3
  Mux2 : Mux  Inputs=3
  Trigonometric Function : Trigonometry  Operator=cos
  Trigonometric Function1 : Trigonometry
  Trigonometric Function2 : Trigonometry
  Trigonometric Function3 : Trigonometry  Operator=cos
  3Rot_Matrix_y : Outport  VectorParamsAs1DForOutWhenUnconnected=off
  wires:
  Matrix Concatenate/1 -> 3Rot_Matrix_y/1
  Constant7/1 -> Mux2/2
  Trigonometric Function2/1 -> Mux/3
  Trigonometric Function/1 -> Mux/1
  Constant8/1 -> Mux/2
  alpha3/1 -> Trigonometric Function/1, Trigonometric Function2/1, Trigonometric Function3/1, Trigonometric Function1/1
  Constant/1 -> Mux1/1
  Constant1/1 -> Mux1/2
  Constant2/1 -> Mux1/3
  Trigonometric Function1/1 -> Gain1/1
  Trigonometric Function3/1 -> Mux2/3
  Mux/1 -> Matrix Concatenate/1
  Mux1/1 -> Matrix Concatenate/2
  Mux2/1 -> Matrix Concatenate/3
  Gain1/1 -> Mux2/1

== system lib_FDM/FDM/FDM_Sophisticated/propulsion/prp_uncertainty/3_rot_mat/3. Rotation z-Achse ==
  alpha3 : Inport
  Constant{4,7..8,10} (4 alike) : Constant  Value=0
  Constant11 : Constant
  Gain : Gain  Gain=-1
  Matrix Concatenate : Concatenate  NumInputs=3  Mode=Multidimensional array  ConcatenateDimension=2
  Mux : Mux  Inputs=3
  Mux1 : Mux  Inputs=3
  Mux2 : Mux  Inputs=3
  Trigonometric Function : Trigonometry  Operator=cos
  Trigonometric Function1 : Trigonometry
  Trigonometric Function3 : Trigonometry  Operator=cos
  Trigonometric Function4 : Trigonometry
  3Rot_Matrix_z : Outport  VectorParamsAs1DForOutWhenUnconnected=off
  wires:
  alpha3/1 -> Trigonometric Function1/1, Trigonometric Function/1, Trigonometric Function4/1, Trigonometric Function3/1
  Matrix Concatenate/1 -> 3Rot_Matrix_z/1
  Constant8/1 -> Mux/3
  Trigonometric Function4/1 -> Gain/1
  Trigonometric Function3/1 -> Mux/1
  Constant11/1 -> Mux2/3
  Constant10/1 -> Mux2/2
  Constant4/1 -> Mux2/1
  Constant7/1 -> Mux1/3
  Trigonometric Function1/1 -> Mux1/1
  Mux2/1 -> Matrix Concatenate/3
  Mux1/1 -> Matrix Concatenate/2
  Mux/1 -> Matrix Concatenate/1
  Trigonometric Function/1 -> Mux1/2
  Gain/1 -> Mux/2

== system lib_FDM/FDM/FDM_Sophisticated/rb_eom/calc_bus_flight_dyn_bus_entries/Subsystem2/trafo_E_to_geodetic ==
  note: Inputs [size]:
      |
      | position_E [3]
  note: Outputs [size]:
      |
      | geodetic longitude [1]
      | geodetic latitude [1]
      | geodetic altitude [1]
  pBEE : Inport
  Geodetic_altitude : Subsystem
  Geodetic_latitude : Subsystem
  Selector1 : Selector  IndexMode=Zero-based  InputPortWidth=3  IndexOptions=Index vector (dialog)  Indices=1  OutputSizes=1
  Selector2 : Selector  IndexMode=Zero-based  InputPortWidth=3  IndexOptions=Index vector (dialog)  Indices=0  OutputSizes=1
  Trigonometric Function1 : Trigonometry  Operator=atan2
  c_flat : Constant  Value=c_flat
  c_rsma : Constant  Value=c_rsma
  lon : Outport  VectorParamsAs1DForOutWhenUnconnected=off
  lat : Outport  Port=2  VectorParamsAs1DForOutWhenUnconnected=off
  alt : Outport  Port=3  VectorParamsAs1DForOutWhenUnconnected=off
  wires:
  pBEE/1 -> Geodetic_altitude/1(pBEE), Geodetic_latitude/1(pBEE), Selector2/1, Selector1/1  "pBEE"
  Trigonometric Function1/1 -> lon/1  "lon"
  Geodetic_altitude/1(alt) -> alt/1
  Geodetic_latitude/1(lat) -> lat/1, Geodetic_altitude/4(lat)
  Selector2/1 -> Trigonometric Function1/2  "pBEE_x"
  Selector1/1 -> Trigonometric Function1/1  "pBEE_y"
  c_rsma/1 -> Geodetic_altitude/2(c_rsma), Geodetic_latitude/2(c_rsma)  "c_rsma"
  c_flat/1 -> Geodetic_latitude/3(c_flat), Geodetic_altitude/3(c_flat)  "c_flat"

== system lib_FDM/FDM/FDM_Sophisticated/rb_eom/eom_6dof/Rigid_Body_EOM_6_DOF/Integration ==
  d_pBII : Inport
  d_vBII : Inport  Port=2
  d_qIB : Inport  Port=3
  d_wBIB : Inport  Port=4
  x0 : Inport  Port=5
  Bus Creator : BusCreator  Inputs=6
  Reshape : Reshape  OutputDimensionality=Customize  OutputDimensions=[13,1]
  Reshape1 : Reshape  OutputDimensionality=Customize  OutputDimensions=[3,1]
  Reshape2 : Reshape  OutputDimensionality=Customize  OutputDimensions=[3,1]
  Selector : Selector  IndexMode=Zero-based  InputPortWidth=13  IndexOptions=Index vector (dialog)  Indices=0:2  OutputSizes=3
  Selector1 : Selector  IndexMode=Zero-based  InputPortWidth=13  IndexOptions=Index vector (dialog)  Indices=3:5  OutputSizes=3
  Selector2 : Selector  IndexMode=Zero-based  InputPortWidth=13  IndexOptions=Index vector (dialog)  Indices=6:9  OutputSizes=3
  Selector3 : Selector  IndexMode=Zero-based  InputPortWidth=13  IndexOptions=Index vector (dialog)  Indices=10:12  OutputSizes=3
  Vector Concatenate : Concatenate  NumInputs=4  ConcatenateDimension=2
  integration_eom : Integrator  InitialConditionSource=external
  normalize_quaternion : Subsystem
      mask help: normalize a quaternion
      mask Help:
      | Name:
      | 
      |     normalize_quaternion
      | 
      | Description:
      | 
      |     This block normalizes the quaternion q21. It should be used as a
      |     safety measure when computing quaternions.
      | 
      | Inputs  [size] [data type] [unit]:
      | 
      |     attitude quaternion q21  [4] [double] [-]
      | 
      | Outputs  [size] [data type] [unit]:
      | 
      |     normalized attitude quaternion q21  [4] [double] [-]
      mask Display: disp (' norm(q)')
  eom : Outport  VectorParamsAs1DForOutWhenUnconnected=off
  wires:
  Bus Creator/1 -> eom/1  "eom_bus"
  Selector3/1 -> Bus Creator/4  "wBIB"
  Selector2/1 -> normalize_quaternion/1(q)  "qIB"
  Selector1/1 -> Bus Creator/2  "vBII"
  Selector/1 -> Bus Creator/1  "pBII"
  x0/1 -> integration_eom/2
  integration_eom/1 -> Selector1/1, Selector/1, Selector3/1, Selector2/1  "x"
  Vector Concatenate/1 -> Reshape/1  "d_x"
  d_wBIB/1 -> Reshape1/1, Vector Concatenate/4
  d_qIB/1 -> Vector Concatenate/3
  d_vBII/1 -> Reshape2/1, Vector Concatenate/2
  d_pBII/1 -> Vector Concatenate/1
  Reshape/1 -> integration_eom/1  "d_x"
  Reshape1/1 -> Bus Creator/5  "d_wBIB"
  Reshape2/1 -> Bus Creator/6  "d_vBII"
  normalize_quaternion/1(q_normalized) -> Bus Creator/3  "qIB"

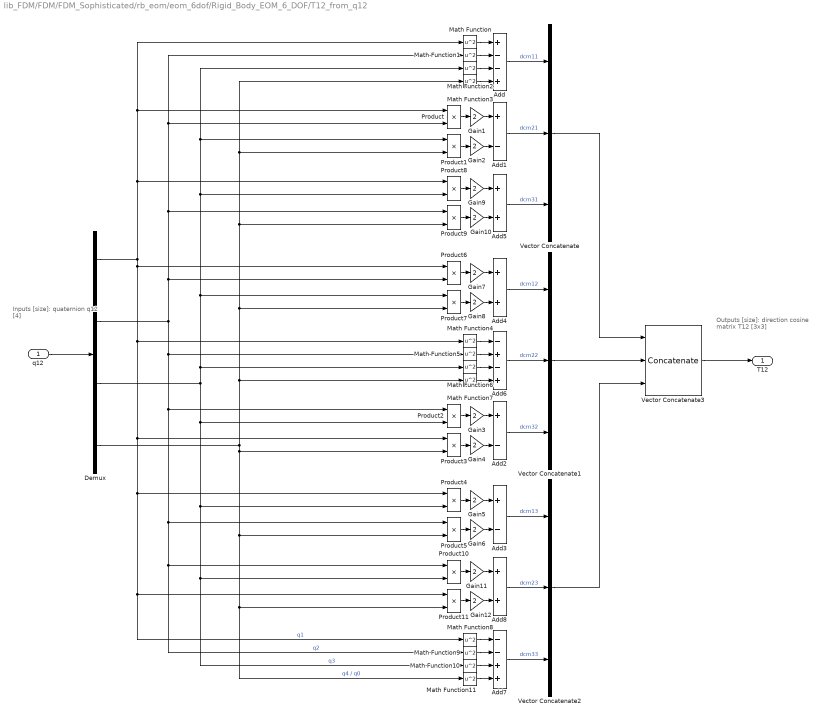
== system lib_FDM/FDM/FDM_Sophisticated/rb_eom/eom_6dof/Rigid_Body_EOM_6_DOF/T12_from_q12 ==
  note: Outputs [size]:
      |
      | direction cosine matrix T12 [3x3]
  note: Inputs [size]:
      |
      | quaternion q12 [4]
  q12 : Inport  PortDimensions=4
  Add : Sum  Inputs=+--+
  Add1 : Sum  Inputs=+-
  Add2 : Sum  Inputs=+-
  Add3 : Sum  Inputs=+-
  Add4 : Sum
  Add5 : Sum
  Add6 : Sum  Inputs=-+-+
  Add7 : Sum  Inputs=--++
  Add8 : Sum
  Demux : Demux
  Gain{1..12} (12 alike) : Gain  Gain=2
  Math Function{,1..11} (12 alike) : Math  Operator=square  SaturateOnIntegerOverflow=on
  Product{,1..11} (12 alike) : Product
  Vector Concatenate : Concatenate  NumInputs=3
  Vector Concatenate1 : Concatenate  NumInputs=3
  Vector Concatenate2 : Concatenate  NumInputs=3
  Vector Concatenate3 : Concatenate  NumInputs=3  Mode=Multidimensional array  ConcatenateDimension=2
  T12 : Outport  PortDimensions=[3 3]  VectorParamsAs1DForOutWhenUnconnected=off
  wires:
  q12/1 -> Demux/1
  Demux/1 -> Product8/1, Product/1, Math Function/1, Product3/1, Product4/1, Product11/1, Math Function8/1, Math Function4/1, Product6/1  "q1"
  Demux/2 -> Product2/1, Product5/1, Product10/1, Math Function9/1, Math Function5/1, Product6/2, Product9/1, Product/2, Math Function1/1  "q2"
  Demux/3 -> Product2/2, Product4/2, Math Function10/1, Product10/2, Math Function6/1, Product7/1, Product8/2, Product1/1, Math Function2/1  "q3"
  Demux/4 -> Math Function7/1, Product7/2, Product9/2, Product1/2, Math Function3/1, Product5/2, Math Function11/1, Product11/2, Product3/2  "q4 / q0"
  Vector Concatenate3/1 -> T12/1
  Vector Concatenate/1 -> Vector Concatenate3/1
  Vector Concatenate2/1 -> Vector Concatenate3/3
  Vector Concatenate1/1 -> Vector Concatenate3/2
  Add/1 -> Vector Concatenate/1  "dcm11"
  Add1/1 -> Vector Concatenate/2  "dcm21"
  Add5/1 -> Vector Concatenate/3  "dcm31"
  Add4/1 -> Vector Concatenate1/1  "dcm12"
  Add6/1 -> Vector Concatenate1/2  "dcm22"
  Add2/1 -> Vector Concatenate1/3  "dcm32"
  Add3/1 -> Vector Concatenate2/1  "dcm13"
  Add8/1 -> Vector Concatenate2/2  "dcm23"
  Add7/1 -> Vector Concatenate2/3  "dcm33"
  Math Function/1 -> Add/1
  Math Function1/1 -> Add/2
  Math Function2/1 -> Add/3
  Math Function3/1 -> Add/4
  Product/1 -> Gain1/1
  Product1/1 -> Gain2/1
  Gain1/1 -> Add1/1
  Gain2/1 -> Add1/2
  Gain4/1 -> Add2/2
  Gain3/1 -> Add2/1
  Product3/1 -> Gain4/1
  Product2/1 -> Gain3/1
  Gain6/1 -> Add3/2
  Gain5/1 -> Add3/1
  Product5/1 -> Gain6/1
  Product4/1 -> Gain5/1
  Gain8/1 -> Add4/2
  Gain7/1 -> Add4/1
  Product7/1 -> Gain8/1
  Product6/1 -> Gain7/1
  Gain10/1 -> Add5/2
  Gain9/1 -> Add5/1
  Product9/1 -> Gain10/1
  Product8/1 -> Gain9/1
  Math Function6/1 -> Add6/3
  Math Function7/1 -> Add6/4
  Math Function5/1 -> Add6/2
  Math Function4/1 -> Add6/1
  Math Function10/1 -> Add7/3
  Math Function11/1 -> Add7/4
  Math Function9/1 -> Add7/2
  Math Function8/1 -> Add7/1
  Gain12/1 -> Add8/2
  Gain11/1 -> Add8/1
  Product11/1 -> Gain12/1
  Product10/1 -> Gain11/1

== system lib_FDM/FDM/FDM_Sophisticated/rb_eom/eom_6dof/Rigid_Body_EOM_6_DOF/rb_eom_6dof ==
  note: d_wBIB = JBB \ (MBTB - d_JBB * wBIB - wBIB x (JBB*wBIB))
  FBTB : Inport
  mB : Inport  Port=2
  JBB : Inport  Port=3
  MBTB : Inport  Port=4
  d_JBB : Inport  Port=5
  qIB : Inport  Port=6
  vBII : Inport  Port=7
  wBIB : Inport  Port=8
  Divide : Product  Inputs=*/
  Divide1 : Product  Inputs=/*  Multiplication=Matrix(*)
  Product : Product  Multiplication=Matrix(*)
  Product1 : Product  Multiplication=Matrix(*)
  Saturation : Saturate  UpperLimit=Inf  LowerLimit=1e-6
      settings: AttributesFormatString=|
      | %<UpperLimit>
      | %<LowerLimit>
  Subtract : Sum  Inputs=+--
  calc_d_qIB : Subsystem
  cross_product : Subsystem
      mask help: cross product r3 = r1 x r2
      mask Help:
      | Name:
      | 
      |     cross_product
      | 
      | Description:
      | 
      |     This block implements the cross product r3 = r1 x r2.
      | 
      | Inputs  [size] [data type] [unit]:
      | 
      |     vector 1  [3] [double] [-]
      |     vector 2  [3] [double] [-]
      | 
      | Outputs  [size] [data type] [unit]:
      | 
      |     resulting vector  [3] [double] [-]
      mask Display: disp(' r3 = r1 x r2')
  r2_from_r1_trans_q21 : Subsystem
      mask help: transforms a vector from frame 1 to frame 2 by a quaternion
      mask Help:
      | Name:
      | 
      |     r2_from_r1_trans_q21
      | 
      | Description:
      | 
      |     This block implements the transformation of a vector from the frame 1
      |     to the frame 2 using the appropriate quaternion.
      | 
      | Inputs  [size] [data type] [unit]:
      | 
      |     vector in frame 1  [3] [double] [-]
      |     attitude quaternion q21  [4] [double] [-]
      | 
      | Outputs  [size] [data type] [unit]:
      | 
      |     vector in frame 2  [3] [double] [-]
      mask Display:
      | port_label('input', 1, 'r1')
      | port_label('input', 2, 'q21')
      | port_label('output', 1, 'r2')
      | disp('r_2 = q_{21} {\bf\cdot} r_1 {\bf\cdot} q_{21}^{\bf\prime}','texmode','on')
  d_pBII : Outport  VectorParamsAs1DForOutWhenUnconnected=off
  d_vBII : Outport  Port=2  VectorParamsAs1DForOutWhenUnconnected=off
  d_qIB : Outport  Port=3  VectorParamsAs1DForOutWhenUnconnected=off
  d_wBIB : Outport  Port=4  VectorParamsAs1DForOutWhenUnconnected=off
  wires:
  FBTB/1 -> Divide/1
  mB/1 -> Saturation/1
  Divide/1 -> r2_from_r1_trans_q21/1(r1)  "aBIB"
  qIB/1 -> r2_from_r1_trans_q21/2(q21), calc_d_qIB/1(qIB)
  r2_from_r1_trans_q21/1(r2) -> d_vBII/1  "aBII"
  vBII/1 -> d_pBII/1
  JBB/1 -> Product1/1, Divide1/1
  wBIB/1 -> Product1/2, cross_product/1(r1), Product/2, calc_d_qIB/2(wBIB)
  Divide1/1 -> d_wBIB/1
  Product/1 -> Subtract/2
  cross_product/1(r1_x_r2) -> Subtract/3
  Product1/1 -> cross_product/2(r2)
  d_JBB/1 -> Product/1
  Subtract/1 -> Divide1/2
  MBTB/1 -> Subtract/1
  calc_d_qIB/1(d_qIB) -> d_qIB/1
  Saturation/1 -> Divide/2

== system lib_FDM/FDM/FDM_Sophisticated/stream_flow/calc_stream_flow/Subsystem1/AoA_Sideslip_Alphatot_Phi ==
  note: falls a_vBEB == 0
      | Alle Winkel = 0
  note: Outputs [size]
      |
      | bus [4]
      | 	al  [1]
      | 	be [1]
      | 	th  [1]
      | 	fi   [1]
  note: Inputs [size]
      |
      | vector vBEB [3]
  vBEB : Inport
  Bus Creator : BusCreator  Inputs=4
  Constant : Constant  Value=[1; 0; 0; 1]
  Demux : Demux
  Demux1 : Demux  Outputs=3
  Divide : Product  Inputs=*/
  Divide1 : Product  Inputs=*/
  Switch : Switch  Criteria=u2 ~= 0
  Trigonometric Function : Trigonometry  Operator=atan2
  Trigonometric Function1 : Trigonometry  Operator=asin
  Trigonometric Function2 : Trigonometry  Operator=acos
  Trigonometric Function3 : Trigonometry  Operator=atan2
  Vector Concatenate : Concatenate  NumInputs=4
  norm_of_vector : Subsystem
      mask help: computes the norm of a vector
      mask Help:
      | Name:
      | 
      |     norm_of_vector
      | 
      | Description:
      | 
      |     This block computes the L2-norm (length) of a vector.
      | 
      | Inputs  [size] [data type] [unit]:
      | 
      |     vector  [3] [double] [-]
      | 
      | Outputs  [size] [data type] [unit]:
      | 
      |     norm of vector  [1] [double] [-]
      mask Display: disp (' norm(r) ')
  aero_angles : Outport  VectorParamsAs1DForOutWhenUnconnected=off
  wires:
  Demux/2 -> Divide/1, Trigonometric Function3/1  "vBEB_y"
  Demux/1 -> Trigonometric Function/2, Divide1/1  "vBEB_x"
  Divide/1 -> Trigonometric Function1/1
  Trigonometric Function/1 -> Bus Creator/1  "al"
  Demux/3 -> Trigonometric Function3/2, Trigonometric Function/1  "vBEB_z"
  vBEB/1 -> Demux1/1, norm_of_vector/1(vector)
  Trigonometric Function1/1 -> Bus Creator/2  "be"
  norm_of_vector/1(norm_of_vector) -> Switch/2, Vector Concatenate/4  "a_vBEB"
  Bus Creator/1 -> aero_angles/1  "aero_angles_bus"
  Constant/1 -> Switch/3
  Vector Concatenate/1 -> Switch/1
  Switch/1 -> Demux/1
  Demux/4 -> Divide/2, Divide1/2  "a_vBEB"
  Trigonometric Function2/1 -> Bus Creator/3  "th"
  Trigonometric Function3/1 -> Bus Creator/4  "fi"
  Divide1/1 -> Trigonometric Function2/1
  Demux1/1 -> Vector Concatenate/1  "vBEB_x"
  Demux1/3 -> Vector Concatenate/3  "vBEB_z"
  Demux1/2 -> Vector Concatenate/2  "vBEB_y"

== system lib_FDM/FDM/FDM_Sophisticated/stream_flow/calc_stream_flow/Subsystem1/calc_nondimensional_rates ==
  a_vB : Inport
  wBIB : Inport  Port=2
  Constant1 : Constant  Value=HIL_Data.FDM.soph.bus1.aero.lref
  Demux : Demux  Outputs=3
  Divide1 : Product  Inputs=/*
  Product2 : Product
  Product3 : Product
  Product4 : Product
  Saturation1 : Saturate  UpperLimit=inf  LowerLimit=100*eps
      settings: AttributesFormatString=|
      | %<UpperLimit>
      | %<LowerLimit>
  Vector Concatenate : Concatenate  NumInputs=3
  wBIB_star : Outport  VectorParamsAs1DForOutWhenUnconnected=off
  wires:
  Vector Concatenate/1 -> wBIB_star/1  "wBIB_star"
  Product2/1 -> Vector Concatenate/1  "pBIB_star"
  Product4/1 -> Vector Concatenate/3  "rBIB_star"
  Constant1/1 -> Divide1/2
  Saturation1/1 -> Divide1/1
  Demux/1 -> Product2/2
  Product3/1 -> Vector Concatenate/2  "qBIB_star"
  wBIB/1 -> Demux/1
  a_vB/1 -> Saturation1/1
  Demux/3 -> Product4/2
  Divide1/1 -> Product2/1, Product3/1, Product4/1
  Demux/2 -> Product3/2

== system lib_FDM/FDM/FDM_Sophisticated/stream_flow/calc_stream_flow/Subsystem1/norm_of_vector ==
  note: Inputs [size]:
      |
      | vector  [3]
  note: Outputs [size]:
      |
      | norm of vector [1]
  vector : Inport
  Dot Product1 : DotProduct  InputSameDT=on  OutDataTypeStr=Inherit: Inherit via internal rule
  Math Function1 : Math  Operator=sqrt  SaturateOnIntegerOverflow=on
  norm_of_vector : Outport  VectorParamsAs1DForOutWhenUnconnected=off
  wires:
  Dot Product1/1 -> Math Function1/1
  Math Function1/1 -> norm_of_vector/1
  vector/1 -> Dot Product1/2, Dot Product1/1
